simulink model "controller"  (Simulink 8.3)
settings: Solver=FixedStepDiscrete  StartTime=0.0  StopTime=inf  FixedStep=CONFIG.TS  RelTol=1e-3
InitFcn:
  | clc
  | cd(fileparts(which(bdroot)));
  | initTrqBalancingSeeSaw;
values from neighbouring files (symbols this model uses):
  LEFT_RIGHT_FOOT_IN_CONTACT = [1;1]    [initTrqBalancingSeeSaw.m]
undefined symbols (not defined in the file or in its folder): bVectorConstraints, CONFIG, ConstraintsMatrix, directionOfOscillation, DiscIntNeverNeededParam, gain, noOscillationTime, referenceParams, reg, ROBOT_DOF, sat, seesaw
undefined symbols (not defined in the file): FRAMES
libraries: WBToolboxLibrary x43
settings Model: Creator=makaveli  LastModifiedBy=gabri
settings DataIOCC: SignalLoggingSaveFormat=Dataset
settings DebuggingCC: UnderspecifiedInitializationDetection=Simplified  MergeDetectMultiDrivingBlocksExec=error  FrameProcessingCompatibilityMsg=error  StateNameClashWarn=none
settings GRTTargetCC: CombineOutputUpdateFcns=on  GRTInterface=off
settings ConfigComp: CovMetricSettings=dw  CovHtmlReporting=on  CovSaveCumulativeToWorkspaceVar=on  CovSaveSingleToWorkspaceVar=on  CovExternalEMLEnable=off  CovSFcnEnable=off

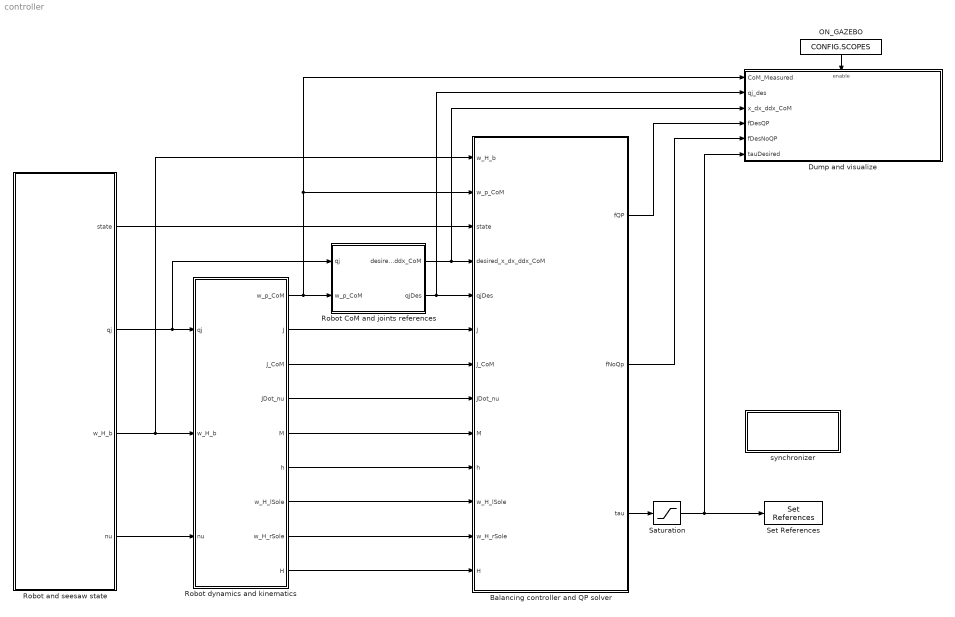
== system controller ==
  Balancing controller and QP solver : Subsystem
  Dump and visualize : Subsystem
  "ON_GAZEBO " : Constant  Value=CONFIG.SCOPES
  Robot CoM and joints references : Subsystem  Priority=2
  Robot and seesaw state : Subsystem
  Robot dynamics and kinematics : Subsystem  Priority=3
  Saturation : Saturate  UpperLimit=sat.torque  LowerLimit=-sat.torque
  Set References : WBToolboxLibrary/wholeBodyActuators/Set References  controlType=Torque  fullOrSubControl=Full  controlledJoints=''  robotName=WBT_robotName  localName=WBT_modelName  wbiFile=WBT_wbiFilename  wbiList=WBT_wbiList
  synchronizer : Subsystem
      mask Display: disp('SYNCHRONIZER')
  wires:
  Robot and seesaw state/1(state) -> Balancing controller and QP solver/3(state)
  Robot CoM and joints references/2(qjDes) -> Dump and visualize/2(qj_des), Balancing controller and QP solver/5(qjDes)
  Robot CoM and joints references/1(desired_x_dx_ddx_CoM) -> Dump and visualize/3(x_dx_ddx_CoM), Balancing controller and QP solver/4(desired_x_dx_ddx_CoM)
  Robot and seesaw state/4(nu) -> Robot dynamics and kinematics/3(nu)
  Robot and seesaw state/2(qj) -> Robot CoM and joints references/1(qj), Robot dynamics and kinematics/1(qj)
  Robot dynamics and kinematics/1(w_p_CoM) -> Balancing controller and QP solver/2(w_p_CoM), Dump and visualize/1(CoM_Measured), Robot CoM and joints references/2(w_p_CoM)
  Robot dynamics and kinematics/2("J ") -> Balancing controller and QP solver/6(J)
  Robot dynamics and kinematics/3(J_CoM) -> Balancing controller and QP solver/7(J_CoM)
  Robot dynamics and kinematics/4(JDot_nu) -> Balancing controller and QP solver/8(JDot_nu)
  Robot dynamics and kinematics/5(M) -> Balancing controller and QP solver/9(M)
  Robot dynamics and kinematics/6(h) -> Balancing controller and QP solver/10(h)
  Robot dynamics and kinematics/7(w_H_lSole) -> Balancing controller and QP solver/11(w_H_lSole)
  Robot dynamics and kinematics/8(w_H_rSole) -> Balancing controller and QP solver/12(w_H_rSole)
  Robot dynamics and kinematics/9(H) -> Balancing controller and QP solver/13(H)
  Balancing controller and QP solver/1(fQP) -> Dump and visualize/4(fDesQP)
  Balancing controller and QP solver/2(fNoQp) -> Dump and visualize/5(fDesNoQP)
  "ON_GAZEBO "/1 -> Dump and visualize/Enable
  Balancing controller and QP solver/3(tau) -> Saturation/1
  Saturation/1 -> Dump and visualize/6(tauDesired), Set References/1
  Robot and seesaw state/3(w_H_b) -> Balancing controller and QP solver/1(w_H_b), Robot dynamics and kinematics/2(w_H_b)

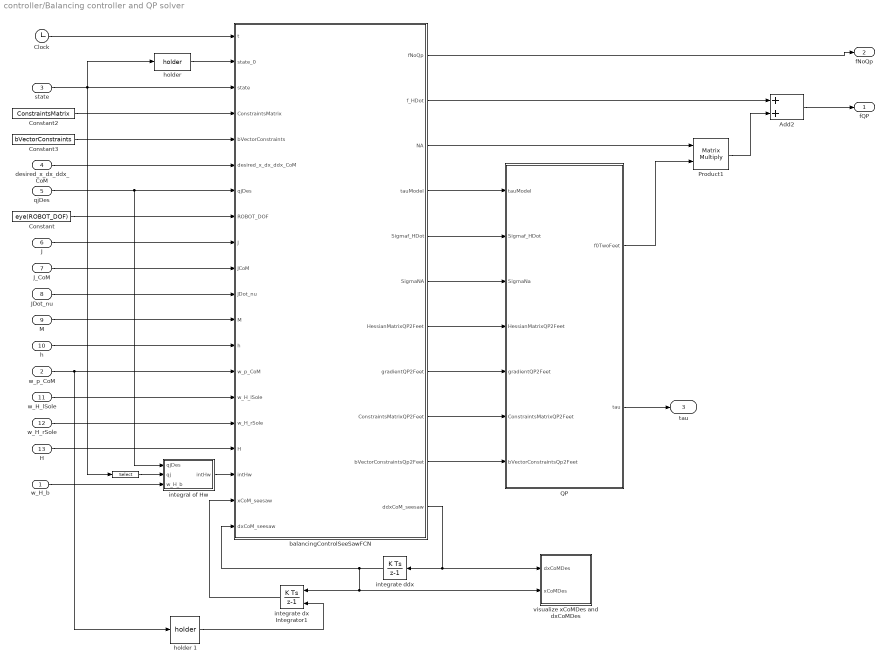
== system controller/Balancing controller and QP solver ==
  w_H_b : Inport
  w_p_CoM : Inport  Port=2
  state : Inport  Port=3
  desired_x_dx_ddx_CoM : Inport  Port=4
  qjDes : Inport  Port=5
  J : Inport  Port=6
  J_CoM : Inport  Port=7
  JDot_nu : Inport  Port=8
  M : Inport  Port=9
  h : Inport  Port=10
  w_H_lSole : Inport  Port=11
  w_H_rSole : Inport  Port=12
  H : Inport  Port=13
  " " : Selector  InputPortWidth=20+2*ROBOT_DOF  Indices=[12:11+ROBOT_DOF]
  Add2 : Sum
  Clock : Clock
  Constant : Constant  Value=eye(ROBOT_DOF)
  Constant2 : Constant  Value=ConstraintsMatrix
  Constant3 : Constant  Value=bVectorConstraints
  Product1 : Product  Multiplication=Matrix(*)
  QP : Subsystem
  balancingControlSeeSawFCN : MATLAB Function  TreatAsAtomicUnit=on
  "holder " : WBToolboxLibrary/Utilities/holder 
  holder 1 : WBToolboxLibrary/Utilities/holder 
  "integral of Hw " : Subsystem
  integrate ddx : DiscreteIntegrator  InitialCondition=zeros(3,1)  SampleTime=CONFIG.TS  ICPrevOutput=DiscIntNeverNeededParam  ICPrevScaledInput=DiscIntNeverNeededParam
  integrate dx Integrator1 : DiscreteIntegrator  InitialConditionSource=external  InitialCondition=zeros(3,1)  SampleTime=CONFIG.TS  ICPrevOutput=DiscIntNeverNeededParam  ICPrevScaledInput=DiscIntNeverNeededParam
  visualize xCoMDes and dxCoMDes : Subsystem
  fQP : Outport
  fNoQp : Outport  Port=2
  tau : Outport  Port=3
  wires:
  Clock/1 -> balancingControlSeeSawFCN/1(t)
  Constant/1 -> balancingControlSeeSawFCN/8(ROBOT_DOF)
  Constant2/1 -> balancingControlSeeSawFCN/4(ConstraintsMatrix)
  Constant3/1 -> balancingControlSeeSawFCN/5(bVectorConstraints)
  QP/1(f0TwoFeet) -> Product1/2
  balancingControlSeeSawFCN/9(ConstraintsMatrixQP2Feet) -> QP/6(ConstraintsMatrixQP2Feet)
  QP/2(tau) -> tau/1
  balancingControlSeeSawFCN/1(fNoQp) -> fNoQp/1
  Product1/1 -> Add2/2
  balancingControlSeeSawFCN/3(NA) -> Product1/1
  balancingControlSeeSawFCN/2(f_HDot) -> Add2/1
  Add2/1 -> fQP/1
  "integral of Hw "/1(intHw) -> balancingControlSeeSawFCN/18(intHw)
  balancingControlSeeSawFCN/4(tauModel) -> QP/1(tauModel)
  balancingControlSeeSawFCN/5(Sigmaf_HDot) -> QP/2(Sigmaf_HDot)
  balancingControlSeeSawFCN/6(SigmaNA) -> QP/3(SigmaNa)
  balancingControlSeeSawFCN/7(HessianMatrixQP2Feet) -> QP/4(HessianMatrixQP2Feet)
  balancingControlSeeSawFCN/8(gradientQP2Feet) -> QP/5(gradientQP2Feet)
  balancingControlSeeSawFCN/10(bVectorConstraintsQp2Feet) -> QP/7(bVectorConstraintsQp2Feet)
  state/1 -> " "/1, balancingControlSeeSawFCN/3(state), "holder "/1
  desired_x_dx_ddx_CoM/1 -> balancingControlSeeSawFCN/6(desired_x_dx_ddx_CoM)
  qjDes/1 -> "integral of Hw "/1(qjDes), balancingControlSeeSawFCN/7(qjDes)
  J/1 -> balancingControlSeeSawFCN/9(J)
  J_CoM/1 -> balancingControlSeeSawFCN/10(JCoM)
  JDot_nu/1 -> balancingControlSeeSawFCN/11(JDot_nu)
  M/1 -> balancingControlSeeSawFCN/12(M)
  h/1 -> balancingControlSeeSawFCN/13(h)
  w_H_lSole/1 -> balancingControlSeeSawFCN/15(w_H_lSole)
  w_H_rSole/1 -> balancingControlSeeSawFCN/16(w_H_rSole)
  H/1 -> balancingControlSeeSawFCN/17(H)
  w_p_CoM/1 -> balancingControlSeeSawFCN/14(w_p_CoM), holder 1/1
  "holder "/1 -> balancingControlSeeSawFCN/2(state_0)
  w_H_b/1 -> "integral of Hw "/3(w_H_b)
  " "/1 -> "integral of Hw "/2(qj)
  balancingControlSeeSawFCN/11(ddxCoM_seesaw) -> integrate ddx/1, visualize xCoMDes and dxCoMDes/1(dxCoMDes)
  integrate dx Integrator1/1 -> balancingControlSeeSawFCN/19(xCoM_seesaw)
  integrate ddx/1 -> integrate dx Integrator1/1, visualize xCoMDes and dxCoMDes/2(xCoMDes), balancingControlSeeSawFCN/20(dxCoM_seesaw)
  holder 1/1 -> integrate dx Integrator1/2

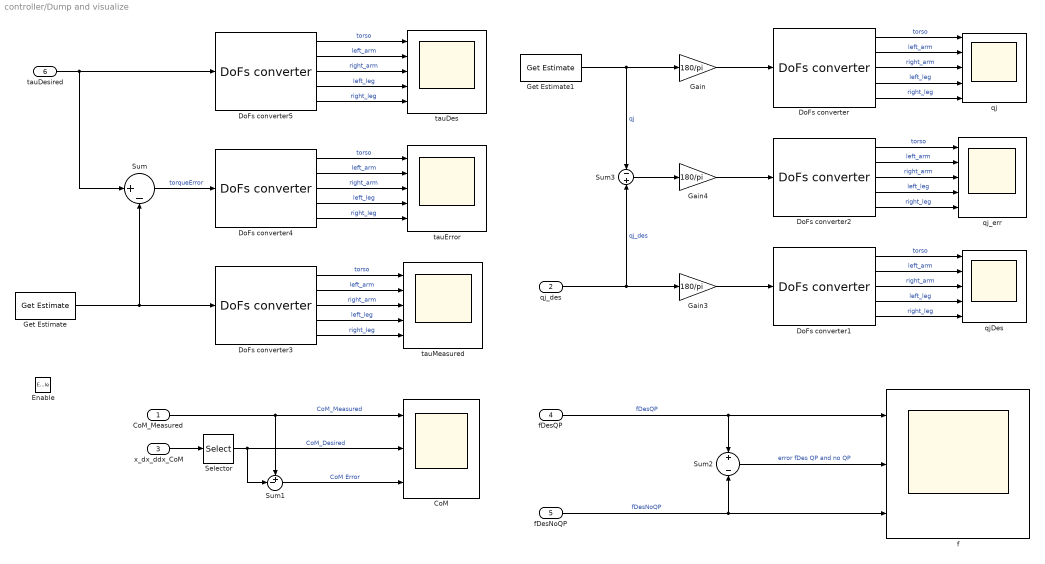
== system controller/Dump and visualize ==
  CoM_Measured : Inport
  qj_des : Inport  Port=2
  x_dx_ddx_CoM : Inport  Port=3
  fDesQP : Inport  Port=4
  fDesNoQP : Inport  Port=5
  tauDesired : Inport  Port=6
  Enable : EnablePort
  CoM : Scope  NumInputPorts=3
      settings: YMin=-5~-5~-5  YMax=5~5~5
  DoFs converter{,1..5} (6 alike) : WBToolboxLibrary/Utilities/DoFs converter  yarp2WBIOption=From WBI to YARP  robotName=WBT_robotName  localName=WBT_modelName  wbiFile=WBT_wbiFilename  wbiList=WBT_wbiList
  Gain : Gain  Gain=180/pi
  Gain3 : Gain  Gain=180/pi
  Gain4 : Gain  Gain=180/pi
  Get Estimate : WBToolboxLibrary/wholeBodyStates/Get Estimate  estimateType=Joints Torque  robotName=WBT_robotName  localName=WBT_modelName  wbiFile=WBT_wbiFilename  wbiList=WBT_wbiList
  Get Estimate1 : WBToolboxLibrary/wholeBodyStates/Get Estimate  estimateType=Joints Position  robotName=WBT_robotName  localName=WBT_modelName  wbiFile=WBT_wbiFilename  wbiList=WBT_wbiList
  Selector : Selector  NumberOfDimensions=2  IndexOptions=Index vector (dialog),Index vector (dialog)  Indices=[1:3],1  OutputSizes=1,1
  Sum : Sum  Inputs=|+-
  Sum1 : Sum  Inputs=+-|
  Sum2 : Sum  Inputs=+|-
  Sum3 : Sum  Inputs=-|+
  f : Scope  NumInputPorts=3
      settings: YMin=-5~-5~-5  YMax=5~5~5
  qj : Scope  NumInputPorts=5
      settings: YMin=-5~-5~-5~-5~-5  YMax=5~5~5~5~5
  qjDes : Scope  NumInputPorts=5
      settings: YMin=-5~-5~-5~-5~-5  YMax=5~5~5~5~5
  qj_err : Scope  NumInputPorts=5
      settings: YMin=-5~-5~-5~-5~-5  YMax=5~5~5~5~5
  tauDes : Scope  NumInputPorts=5
      settings: YMin=-5~-5~-5~-5~-5  YMax=5~5~5~5~5
  tauError : Scope  NumInputPorts=5
      settings: YMin=-5~-5~-5~-5~-5  YMax=5~5~5~5~5
  tauMeasured : Scope  NumInputPorts=5
      settings: YMin=-5~-5~-5~-5~-5  YMax=5~5~5~5~5
  wires:
  x_dx_ddx_CoM/1 -> Selector/1
  CoM_Measured/1 -> Sum1/1, CoM/1  "CoM_Measured"
  Get Estimate1/1 -> Sum3/1, Gain/1  "qj"
  Gain/1 -> DoFs converter/1
  DoFs converter/5 -> qj/5  "right_leg"
  DoFs converter/1 -> qj/1  "torso"
  DoFs converter/2 -> qj/2  "left_arm"
  DoFs converter/4 -> qj/4  "left_leg"
  DoFs converter/3 -> qj/3  "right_arm"
  fDesQP/1 -> Sum2/1, f/1  "fDesQP"
  Sum2/1 -> f/2  "error fDes QP and no QP"
  fDesNoQP/1 -> Sum2/2, f/3  "fDesNoQP"
  tauDesired/1 -> DoFs converter5/1, Sum/1
  Get Estimate/1 -> Sum/2, DoFs converter3/1
  DoFs converter5/5 -> tauDes/5  "right_leg"
  DoFs converter5/1 -> tauDes/1  "torso"
  DoFs converter5/2 -> tauDes/2  "left_arm"
  DoFs converter5/4 -> tauDes/4  "left_leg"
  DoFs converter5/3 -> tauDes/3  "right_arm"
  DoFs converter4/5 -> tauError/5  "right_leg"
  DoFs converter4/1 -> tauError/1  "torso"
  DoFs converter4/2 -> tauError/2  "left_arm"
  DoFs converter4/4 -> tauError/4  "left_leg"
  DoFs converter4/3 -> tauError/3  "right_arm"
  Sum/1 -> DoFs converter4/1  "torqueError"
  DoFs converter3/5 -> tauMeasured/5  "right_leg"
  DoFs converter3/1 -> tauMeasured/1  "torso"
  DoFs converter3/2 -> tauMeasured/2  "left_arm"
  DoFs converter3/4 -> tauMeasured/4  "left_leg"
  DoFs converter3/3 -> tauMeasured/3  "right_arm"
  qj_des/1 -> Sum3/2, Gain3/1  "qj_des"
  Gain3/1 -> DoFs converter1/1
  DoFs converter1/5 -> qjDes/5  "right_leg"
  DoFs converter1/1 -> qjDes/1  "torso"
  DoFs converter1/2 -> qjDes/2  "left_arm"
  DoFs converter1/4 -> qjDes/4  "left_leg"
  DoFs converter1/3 -> qjDes/3  "right_arm"
  Gain4/1 -> DoFs converter2/1
  DoFs converter2/5 -> qj_err/5  "right_leg"
  DoFs converter2/1 -> qj_err/1  "torso"
  DoFs converter2/2 -> qj_err/2  "left_arm"
  DoFs converter2/4 -> qj_err/4  "left_leg"
  DoFs converter2/3 -> qj_err/3  "right_arm"
  Sum3/1 -> Gain4/1
  Selector/1 -> Sum1/2, CoM/2  "CoM_Desired"
  Sum1/1 -> CoM/3  "CoM Error"

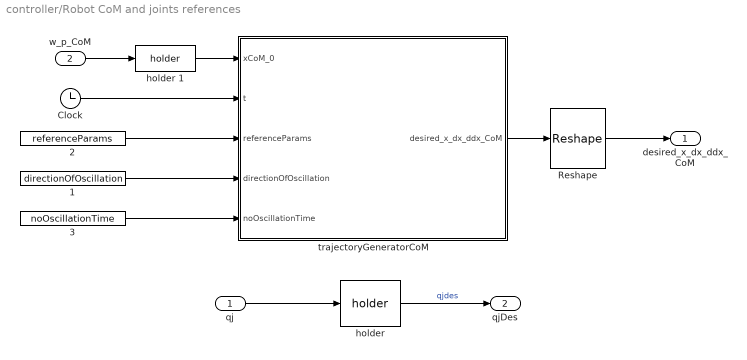
== system controller/Robot CoM and joints references ==
  qj : Inport
  w_p_CoM : Inport  Port=2
  "    1" : Constant  Value=directionOfOscillation
  "    2" : Constant  Value=referenceParams
  "    3" : Constant  Value=noOscillationTime
  Clock : Clock
  Reshape : Reshape  OutputDimensionality=Customize  OutputDimensions=[3,3]
  "holder " : WBToolboxLibrary/Utilities/holder 
  holder 1 : WBToolboxLibrary/Utilities/holder 
  trajectoryGeneratorCoM : MATLAB Function  TreatAsAtomicUnit=on
  desired_x_dx_ddx_CoM : Outport
  qjDes : Outport  Port=2
  wires:
  qj/1 -> "holder "/1
  "holder "/1 -> qjDes/1  "qjdes"
  holder 1/1 -> trajectoryGeneratorCoM/1(xCoM_0)
  "    2"/1 -> trajectoryGeneratorCoM/3(referenceParams)
  Clock/1 -> trajectoryGeneratorCoM/2(t)
  "    1"/1 -> trajectoryGeneratorCoM/4(directionOfOscillation)
  "    3"/1 -> trajectoryGeneratorCoM/5(noOscillationTime)
  trajectoryGeneratorCoM/1(desired_x_dx_ddx_CoM) -> Reshape/1
  Reshape/1 -> desired_x_dx_ddx_CoM/1
  w_p_CoM/1 -> holder 1/1

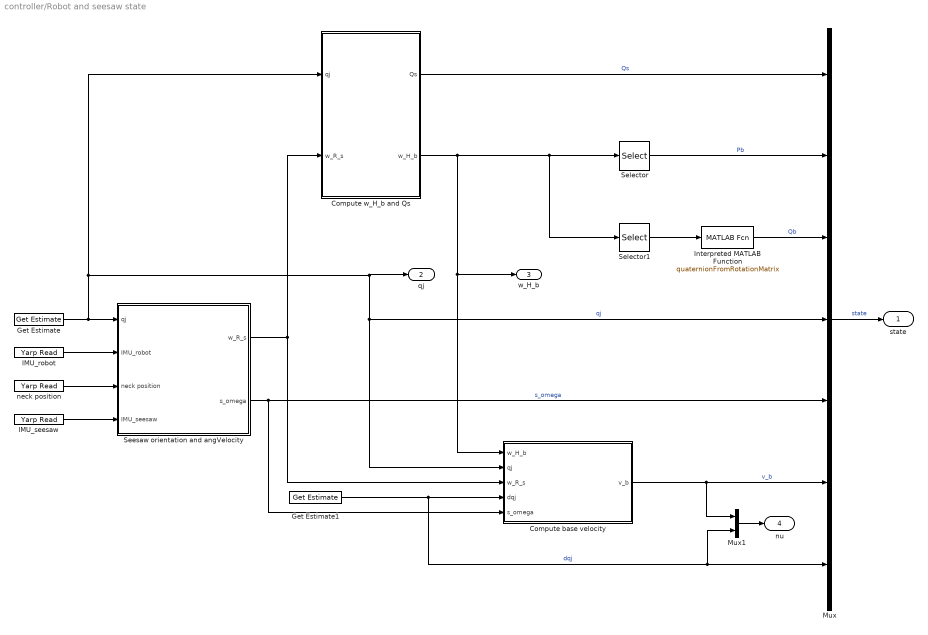
== system controller/Robot and seesaw state ==
  Compute base velocity : Subsystem
  "Compute w_H_b and Qs " : Subsystem
  Get Estimate : WBToolboxLibrary/wholeBodyStates/Get Estimate  estimateType=Joints Position  robotName=WBT_robotName  localName=WBT_modelName  wbiFile=WBT_wbiFilename  wbiList=WBT_wbiList
  Get Estimate1 : WBToolboxLibrary/wholeBodyStates/Get Estimate  estimateType=Joints Velocity  robotName=WBT_robotName  localName=WBT_modelName  wbiFile=WBT_wbiFilename  wbiList=WBT_wbiList
  IMU_robot : WBToolboxLibrary/Utilities/Yarp Read  portName=PORTS.IMU  signalSize=12  blocking=off  timestamp=off  autoconnect=on  errorOnConnection=on
  IMU_seesaw : WBToolboxLibrary/Utilities/Yarp Read  portName=PORTS.IMU_SEESAW  signalSize=12  blocking=off  timestamp=off  autoconnect=on  errorOnConnection=off
  Interpreted MATLAB Function : MATLABFcn  MATLABFcn=quaternionFromRotationMatrix  OutputDimensions=4
  Mux : Mux  Inputs=7
  Mux1 : Mux  Inputs=2
  Seesaw orientation and angVelocity : Subsystem
  Selector : Selector  NumberOfDimensions=2  InputPortWidth=3  IndexOptions=Index vector (dialog),Index vector (dialog)  Indices=[1:3],4  OutputSizes=1,1
  Selector1 : Selector  NumberOfDimensions=2  InputPortWidth=3  IndexOptions=Index vector (dialog),Index vector (dialog)  Indices=[1:3],[1:3]  OutputSizes=1,1
  neck position : WBToolboxLibrary/Utilities/Yarp Read  portName=PORTS.NECK  signalSize=6  blocking=off  timestamp=off  autoconnect=on  errorOnConnection=on
  state : Outport
  qj : Outport  Port=2
  w_H_b : Outport  Port=3
  nu : Outport  Port=4
  wires:
  IMU_robot/1 -> Seesaw orientation and angVelocity/2(IMU_robot)
  IMU_seesaw/1 -> Seesaw orientation and angVelocity/4(IMU_seesaw)
  neck position/1 -> Seesaw orientation and angVelocity/3(neck position)
  Mux/1 -> state/1  "state"
  Selector/1 -> Mux/2  "Pb"
  Selector1/1 -> Interpreted MATLAB Function/1
  Interpreted MATLAB Function/1 -> Mux/3  "Qb"
  Get Estimate/1 -> "Compute w_H_b and Qs "/1(qj), qj/1, Compute base velocity/2(qj), Mux/4, Seesaw orientation and angVelocity/1(qj)  "qj"
  Mux1/1 -> nu/1
  Compute base velocity/1(v_b) -> Mux1/1, Mux/6  "v_b"
  Seesaw orientation and angVelocity/1(w_R_s) -> "Compute w_H_b and Qs "/2(w_R_s), Compute base velocity/3(w_R_s)
  Seesaw orientation and angVelocity/2(s_omega) -> Mux/5, Compute base velocity/5(s_omega)  "s_omega"
  Get Estimate1/1 -> Mux1/2, Mux/7, Compute base velocity/4(dqj)  "dqj"
  "Compute w_H_b and Qs "/2(w_H_b) -> w_H_b/1, Compute base velocity/1(w_H_b), Selector1/1, Selector/1
  "Compute w_H_b and Qs "/1(Qs) -> Mux/1  "Qs"

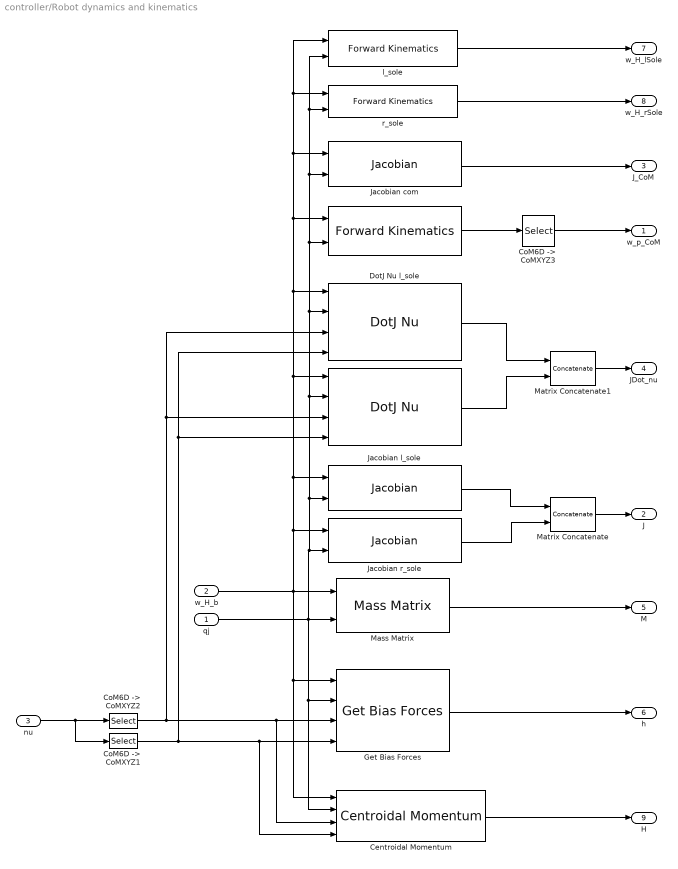
== system controller/Robot dynamics and kinematics ==
  qj : Inport
  w_H_b : Inport  Port=2
  nu : Inport  Port=3
  " " : WBToolboxLibrary/wholeBodyModel/Kinematics/Forward Kinematics  frameName='com'  robotName=WBT_robotName  localName=WBT_modelName  wbiFile=WBT_wbiFilename  wbiList=WBT_wbiList
  "  " : WBToolboxLibrary/wholeBodyModel/Jacobians/DotJ Nu  frameName='r_sole'  robotName=WBT_robotName  localName=WBT_modelName  wbiFile=WBT_wbiFilename  wbiList=WBT_wbiList
  Centroidal Momentum : WBToolboxLibrary/wholeBodyModel/Dynamics/Centroidal Momentum  robotName=WBT_robotName  localName=WBT_modelName  wbiFile=WBT_wbiFilename  wbiList=WBT_wbiList
  "CoM6D ->  CoMXYZ1" : Selector  InputPortWidth=6+ROBOT_DOF  Indices=[7:6+ROBOT_DOF]
  "CoM6D ->  CoMXYZ2" : Selector  InputPortWidth=6+ROBOT_DOF  Indices=[1 2 3 4 5 6]
  "CoM6D ->  CoMXYZ3" : Selector  NumberOfDimensions=2  InputPortWidth=7  IndexOptions=Index vector (dialog),Index vector (dialog)  Indices=[1 2 3],[4]  OutputSizes=1,1
  "DotJ Nu l_sole " : WBToolboxLibrary/wholeBodyModel/Jacobians/DotJ Nu  frameName='l_sole'  robotName=WBT_robotName  localName=WBT_modelName  wbiFile=WBT_wbiFilename  wbiList=WBT_wbiList
  Get Bias Forces : WBToolboxLibrary/wholeBodyModel/Dynamics/Get Bias Forces  robotName=WBT_robotName  localName=WBT_modelName  wbiFile=WBT_wbiFilename  wbiList=WBT_wbiList  explicitGravity=off
  Jacobian com : WBToolboxLibrary/wholeBodyModel/Jacobians/Jacobian  frameName='com'  robotName=WBT_robotName  localName=WBT_modelName  wbiFile=WBT_wbiFilename  wbiList=WBT_wbiList
  Jacobian l_sole : WBToolboxLibrary/wholeBodyModel/Jacobians/Jacobian  frameName='l_sole'  robotName=WBT_robotName  localName=WBT_modelName  wbiFile=WBT_wbiFilename  wbiList=WBT_wbiList
  Jacobian r_sole : WBToolboxLibrary/wholeBodyModel/Jacobians/Jacobian  frameName='r_sole'  robotName=WBT_robotName  localName=WBT_modelName  wbiFile=WBT_wbiFilename  wbiList=WBT_wbiList
  Mass Matrix : WBToolboxLibrary/wholeBodyModel/Dynamics/Mass Matrix  robotName=WBT_robotName  localName=WBT_modelName  wbiFile=WBT_wbiFilename  wbiList=WBT_wbiList
  Matrix Concatenate : Concatenate  Mode=Multidimensional array
  Matrix Concatenate1 : Concatenate  Mode=Multidimensional array
  l_sole : WBToolboxLibrary/wholeBodyModel/Kinematics/Forward Kinematics  frameName='l_sole'  robotName=WBT_robotName  localName=WBT_modelName  wbiFile=WBT_wbiFilename  wbiList=WBT_wbiList
  r_sole : WBToolboxLibrary/wholeBodyModel/Kinematics/Forward Kinematics  frameName='r_sole'  robotName=WBT_robotName  localName=WBT_modelName  wbiFile=WBT_wbiFilename  wbiList=WBT_wbiList
  w_p_CoM : Outport
  "J " : Outport  Port=2
  J_CoM : Outport  Port=3
  JDot_nu : Outport  Port=4
  M : Outport  Port=5
  h : Outport  Port=6
  w_H_lSole : Outport  Port=7
  w_H_rSole : Outport  Port=8
  H : Outport  Port=9
  wires:
  Get Bias Forces/1 -> h/1
  Matrix Concatenate1/1 -> JDot_nu/1
  Jacobian r_sole/1 -> Matrix Concatenate/2
  l_sole/1 -> w_H_lSole/1
  r_sole/1 -> w_H_rSole/1
  Matrix Concatenate/1 -> "J "/1
  Jacobian l_sole/1 -> Matrix Concatenate/1
  Jacobian com/1 -> J_CoM/1
  w_H_b/1 -> Jacobian r_sole/1, "  "/1, " "/1, r_sole/1, l_sole/1, Jacobian com/1, "DotJ Nu l_sole "/1, Jacobian l_sole/1, Mass Matrix/1, Centroidal Momentum/1, Get Bias Forces/1
  qj/1 -> Centroidal Momentum/2, Get Bias Forces/2, r_sole/2, l_sole/2, Jacobian com/2, " "/2, "DotJ Nu l_sole "/2, "  "/2, Jacobian l_sole/2, Jacobian r_sole/2, Mass Matrix/2
  "CoM6D ->  CoMXYZ2"/1 -> "  "/3, "DotJ Nu l_sole "/3, Centroidal Momentum/3, Get Bias Forces/3
  "CoM6D ->  CoMXYZ1"/1 -> Centroidal Momentum/4, Get Bias Forces/4, "  "/4, "DotJ Nu l_sole "/4
  nu/1 -> "CoM6D ->  CoMXYZ1"/1, "CoM6D ->  CoMXYZ2"/1
  Centroidal Momentum/1 -> H/1
  Mass Matrix/1 -> M/1
  "DotJ Nu l_sole "/1 -> Matrix Concatenate1/1
  "  "/1 -> Matrix Concatenate1/2
  "CoM6D ->  CoMXYZ3"/1 -> w_p_CoM/1
  " "/1 -> "CoM6D ->  CoMXYZ3"/1

== system controller/synchronizer ==
  GAZEBO_SYNCHRONIZER : Subsystem
  Logical Operator : Logic  Operator=NOT  AllPortsSameDT=off  OutDataTypeStr=boolean
  "ON_GAZEBO " : Constant  Value=CONFIG.ON_GAZEBO
  REAL_TIME_SYNC : Subsystem
  wires:
  Logical Operator/1 -> REAL_TIME_SYNC/Enable
  "ON_GAZEBO "/1 -> Logical Operator/1, GAZEBO_SYNCHRONIZER/Enable

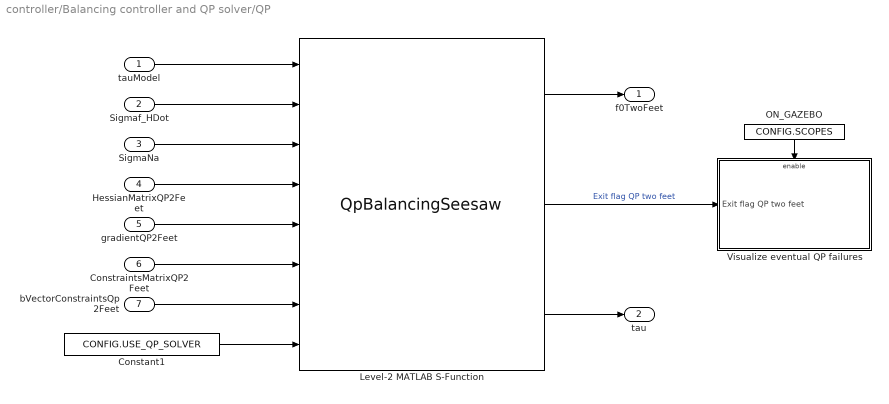
== system controller/Balancing controller and QP solver/QP ==
  tauModel : Inport
  Sigmaf_HDot : Inport  Port=2
  SigmaNa : Inport  Port=3
  HessianMatrixQP2Feet : Inport  Port=4
  gradientQP2Feet : Inport  Port=5
  ConstraintsMatrixQP2Feet : Inport  Port=6
  bVectorConstraintsQp2Feet : Inport  Port=7
  Constant1 : Constant  Value=CONFIG.USE_QP_SOLVER
  Level-2 MATLAB S-Function : M-S-Function  FunctionName=QpBalancingSeesaw
  "ON_GAZEBO " : Constant  Value=CONFIG.SCOPES
  Visualize eventual QP failures : Subsystem
  f0TwoFeet : Outport
  tau : Outport  Port=2
  wires:
  Level-2 MATLAB S-Function/1 -> f0TwoFeet/1
  Level-2 MATLAB S-Function/2 -> Visualize eventual QP failures/1(Exit flag QP two feet)  "Exit flag QP two feet"
  "ON_GAZEBO "/1 -> Visualize eventual QP failures/Enable
  Constant1/1 -> Level-2 MATLAB S-Function/8
  HessianMatrixQP2Feet/1 -> Level-2 MATLAB S-Function/4
  gradientQP2Feet/1 -> Level-2 MATLAB S-Function/5
  ConstraintsMatrixQP2Feet/1 -> Level-2 MATLAB S-Function/6
  bVectorConstraintsQp2Feet/1 -> Level-2 MATLAB S-Function/7
  tauModel/1 -> Level-2 MATLAB S-Function/1
  Sigmaf_HDot/1 -> Level-2 MATLAB S-Function/2
  SigmaNa/1 -> Level-2 MATLAB S-Function/3
  Level-2 MATLAB S-Function/3 -> tau/1

== system controller/Balancing controller and QP solver/integral of Hw  ==
  qjDes : Inport
  qj : Inport  Port=2
  w_H_b : Inport  Port=3
  "  " : WBToolboxLibrary/wholeBodyModel/Jacobians/Jacobian  frameName='r_sole'  robotName=WBT_robotName  localName=WBT_modelName  wbiFile=WBT_wbiFilename  wbiList=WBT_wbiList
  Centroidal Momentum : WBToolboxLibrary/wholeBodyModel/Dynamics/Centroidal Momentum  robotName=WBT_robotName  localName=WBT_modelName  wbiFile=WBT_wbiFilename  wbiList=WBT_wbiList
  Constant4 : Constant  Value=LEFT_RIGHT_FOOT_IN_CONTACT
  Jacobian : WBToolboxLibrary/wholeBodyModel/Jacobians/Jacobian  frameName='l_sole'  robotName=WBT_robotName  localName=WBT_modelName  wbiFile=WBT_wbiFilename  wbiList=WBT_wbiList
  MATLAB Function : MATLAB Function  TreatAsAtomicUnit=on
  Selector : Selector  InputPortWidth=6  Indices=[4 5 6]
  Sum : Sum  Inputs=|-+
  "holder " : WBToolboxLibrary/Utilities/holder 
  intHw : Outport
  wires:
  qjDes/1 -> Sum/1, "  "/2, Jacobian/2, Centroidal Momentum/2
  qj/1 -> Sum/2
  Sum/1 -> MATLAB Function/1(qjErr), Centroidal Momentum/4
  MATLAB Function/1(vbEquivalent) -> Centroidal Momentum/3
  Jacobian/1 -> MATLAB Function/2(JL)
  Centroidal Momentum/1 -> Selector/1
  Selector/1 -> intHw/1
  "  "/1 -> MATLAB Function/3(JR)
  w_H_b/1 -> "holder "/1
  Constant4/1 -> MATLAB Function/4(activeFeetConstraints)
  "holder "/1 -> Centroidal Momentum/1, Jacobian/1, "  "/1

== system controller/Balancing controller and QP solver/visualize xCoMDes and dxCoMDes ==
  dxCoMDes : Inport
  xCoMDes : Inport  Port=2
  vis_dxCoMDes : Scope
      settings: SaveName=ScopeData12
  vis_xCoMDes : Scope
      settings: YMin=-0.011  YMax=0.007  SaveName=ScopeData11
  wires:
  dxCoMDes/1 -> vis_dxCoMDes/1
  xCoMDes/1 -> vis_xCoMDes/1

== system controller/Robot and seesaw state/Compute base velocity ==
  w_H_b : Inport
  qj : Inport  Port=2
  w_R_s : Inport  Port=3
  dqj : Inport  Port=4
  s_omega : Inport  Port=5
  Base and joints velocity : Subsystem
  Jacobian fixedLink : WBToolboxLibrary/wholeBodyModel/Jacobians/Jacobian  frameName=FRAMES.fixedLink  robotName=WBT_robotName  localName=WBT_modelName  wbiFile=WBT_wbiFilename  wbiList=WBT_wbiList
  "ON_GAZEBO " : Constant  Value=CONFIG.SCOPES
  evaluateBaseVelocity : MATLAB Function  Priority=10  TreatAsAtomicUnit=on
  v_b : Outport
  wires:
  w_R_s/1 -> evaluateBaseVelocity/2(w_R_s)
  w_H_b/1 -> Jacobian fixedLink/1
  evaluateBaseVelocity/1(v_base) -> Base and joints velocity/1(v_b), v_b/1
  s_omega/1 -> evaluateBaseVelocity/4(s_omega)
  qj/1 -> Jacobian fixedLink/2
  dqj/1 -> evaluateBaseVelocity/3(dqj), Base and joints velocity/2(dqj)
  Jacobian fixedLink/1 -> evaluateBaseVelocity/1(J_fixedLink)
  "ON_GAZEBO "/1 -> Base and joints velocity/Enable

== system controller/Robot and seesaw state/Compute w_H_b and Qs  ==
  qj : Inport
  w_R_s : Inport  Port=2
  Compute w_H_fixedLink : Subsystem
  MATLAB Function : MATLAB Function  Priority=10  TreatAsAtomicUnit=on
  Product1 : Product  Priority=19  Multiplication=Matrix(*)
  fixedLink_H_b : Subsystem  mask{link_name=FRAMES.fixedLink}
      mask prompts: link_name "link name"
      mask help:
      | This block evaluates the homogeneous transformation between the world and the root link, i.e. ^wH_b. It assumes that the link specified by the variable 'link_name' has a constant position
      | w.r.t. an inertial frame, but it can rotate arbitrarily. This rotation is retrived from the IMU sensor.
      mask Display:
      | str = strrep(link_name, '_','\_');
      | port_label('output',1,['{}^{',str '}H_{root}'],'texmode','on')
      | clear str;
      | 
      | port_label('input',1,'q_j','texmode','on')
  Qs : Outport
  w_H_b : Outport  Port=2
  wires:
  qj/1 -> fixedLink_H_b/1(qj)
  w_R_s/1 -> Compute w_H_fixedLink/1(w_R_s), MATLAB Function/1(w_R_s)
  fixedLink_H_b/1(link_H_root) -> Product1/2
  MATLAB Function/1(Qs) -> Qs/1  "Qs"
  Product1/1 -> w_H_b/1  "w_H_b"
  Compute w_H_fixedLink/1(w_H_fixedLink) -> Product1/1

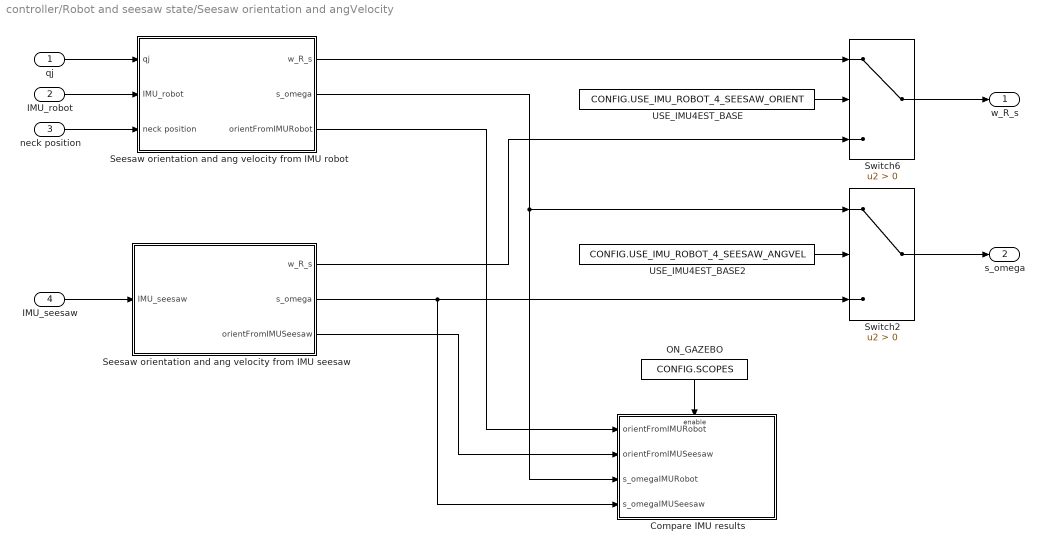
== system controller/Robot and seesaw state/Seesaw orientation and angVelocity ==
  qj : Inport
  IMU_robot : Inport  Port=2
  neck position : Inport  Port=3
  IMU_seesaw : Inport  Port=4
  Compare IMU results : Subsystem
  "ON_GAZEBO " : Constant  Value=CONFIG.SCOPES
  Seesaw orientation and ang velocity from IMU robot : Subsystem
  Seesaw orientation and ang velocity from IMU seesaw : Subsystem
  Switch2 : Switch  Criteria=u2 > Threshold
  Switch6 : Switch  Criteria=u2 > Threshold
  USE_IMU4EST_BASE : Constant  Value=CONFIG.USE_IMU_ROBOT_4_SEESAW_ORIENT
  USE_IMU4EST_BASE2 : Constant  Value=CONFIG.USE_IMU_ROBOT_4_SEESAW_ANGVEL
  w_R_s : Outport
  s_omega : Outport  Port=2
  wires:
  USE_IMU4EST_BASE/1 -> Switch6/2
  Switch6/1 -> w_R_s/1
  Seesaw orientation and ang velocity from IMU seesaw/1(w_R_s) -> Switch6/3
  IMU_seesaw/1 -> Seesaw orientation and ang velocity from IMU seesaw/1(IMU_seesaw)
  Seesaw orientation and ang velocity from IMU robot/1(w_R_s) -> Switch6/1
  neck position/1 -> Seesaw orientation and ang velocity from IMU robot/3(neck position)
  USE_IMU4EST_BASE2/1 -> Switch2/2
  IMU_robot/1 -> Seesaw orientation and ang velocity from IMU robot/2(IMU_robot)
  qj/1 -> Seesaw orientation and ang velocity from IMU robot/1(qj)
  Seesaw orientation and ang velocity from IMU robot/2(s_omega) -> Compare IMU results/3(s_omegaIMURobot), Switch2/1
  Seesaw orientation and ang velocity from IMU seesaw/2(s_omega) -> Compare IMU results/4(s_omegaIMUSeesaw), Switch2/3
  Switch2/1 -> s_omega/1
  Seesaw orientation and ang velocity from IMU robot/3(orientFromIMURobot) -> Compare IMU results/1(orientFromIMURobot)
  Seesaw orientation and ang velocity from IMU seesaw/3(orientFromIMUSeesaw) -> Compare IMU results/2(orientFromIMUSeesaw)
  "ON_GAZEBO "/1 -> Compare IMU results/Enable

== system controller/synchronizer/GAZEBO_SYNCHRONIZER ==
  Enable : EnablePort
  Simulator Synchronizer : WBToolboxLibrary/Utilities/Simulator Synchronizer  period=CONFIG.TS  serverPortName='/clock/rpc'  clientPortName='/WBT_synchronizer/rpc:o'

== system controller/synchronizer/REAL_TIME_SYNC ==
  Enable : EnablePort
  Real Time Synchronizer : WBToolboxLibrary/Utilities/Real Time Synchronizer  period=CONFIG.TS

== system controller/Balancing controller and QP solver/QP/Visualize eventual QP failures ==
  Exit flag QP two feet : Inport
  Enable : EnablePort
  "QP status (0: no failure, 1: not using)" : Scope
  wires:
  Exit flag QP two feet/1 -> "QP status (0: no failure, 1: not using)"/1

== system controller/Robot and seesaw state/Compute base velocity/Base and joints velocity ==
  v_b : Inport
  dqj : Inport  Port=2
  Enable : EnablePort
  DoFs converter : WBToolboxLibrary/Utilities/DoFs converter  yarp2WBIOption=From WBI to YARP  robotName=WBT_robotName  localName=WBT_modelName  wbiFile=WBT_wbiFilename  wbiList=WBT_wbiList
  dq_j : Scope  NumInputPorts=5
      settings: YMin=-5~-5~-5~-5~-5  YMax=5~5~5~5~5  SaveName=ScopeData2
  vb : Scope
      settings: SaveName=ScopeData10
  wires:
  DoFs converter/5 -> dq_j/5  "right_leg"
  DoFs converter/1 -> dq_j/1  "torso"
  DoFs converter/2 -> dq_j/2  "left_arm"
  DoFs converter/4 -> dq_j/4  "left_leg"
  DoFs converter/3 -> dq_j/3  "right_arm"
  dqj/1 -> DoFs converter/1
  v_b/1 -> vb/1

== system controller/Robot and seesaw state/Compute w_H_b and Qs /Compute w_H_fixedLink ==
  w_R_s : Inport
  fixedLink w.r.t the world frame : MATLAB Function  TreatAsAtomicUnit=on
  w_H_fixedLink : Outport
  wires:
  w_R_s/1 -> fixedLink w.r.t the world frame/1(w_R_s)
  fixedLink w.r.t the world frame/1(w_H_fixedLink) -> w_H_fixedLink/1

== system controller/Robot and seesaw state/Compute w_H_b and Qs /fixedLink_H_b ==
  qj : Inport
  Constant2 : Constant  Value=eye(4)
  Constant6 : Constant  Value=eye(4)
  Inv\*1 : Product  Inputs=/*  Multiplication=Matrix(*)
  link : WBToolboxLibrary/wholeBodyModel/Kinematics/Forward Kinematics  frameName=link_name  robotName=WBT_robotName  localName=WBT_modelName  wbiFile=WBT_wbiFilename  wbiList=WBT_wbiList
  root_link : WBToolboxLibrary/wholeBodyModel/Kinematics/Forward Kinematics  frameName='root_link'  robotName=WBT_robotName  localName=WBT_modelName  wbiFile=WBT_wbiFilename  wbiList=WBT_wbiList
  link_H_root : Outport
  wires:
  Constant6/1 -> link/1
  Inv\*1/1 -> link_H_root/1
  link/1 -> Inv\*1/1
  Constant2/1 -> root_link/1
  qj/1 -> root_link/2, link/2
  root_link/1 -> Inv\*1/2

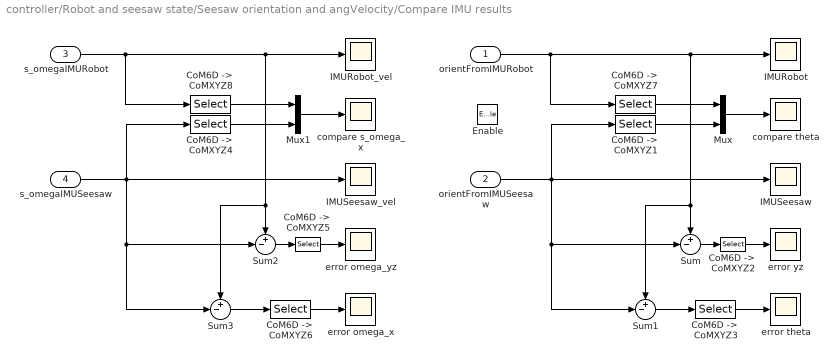
== system controller/Robot and seesaw state/Seesaw orientation and angVelocity/Compare IMU results ==
  orientFromIMURobot : Inport
  orientFromIMUSeesaw : Inport  Port=2
  s_omegaIMURobot : Inport  Port=3
  s_omegaIMUSeesaw : Inport  Port=4
  Enable : EnablePort
  CoM6D ->  CoMXYZ{1,3..4,6..8} (6 alike) : Selector  InputPortWidth=3  Indices=[1]
  "CoM6D ->  CoMXYZ2" : Selector  InputPortWidth=3  Indices=[2 3]
  "CoM6D ->  CoMXYZ5" : Selector  InputPortWidth=3  Indices=[2 3]
  IMURobot : Scope
  IMURobot_vel : Scope
      settings: SaveName=ScopeData5
  IMUSeesaw : Scope
  IMUSeesaw_vel : Scope
      settings: SaveName=ScopeData6
  Mux : Mux  Inputs=2
  Mux1 : Mux  Inputs=2
  Sum{,1..3} (4 alike) : Sum  Inputs=+-|
  compare s_omega_x : Scope
      settings: SaveName=ScopeData7
  compare theta : Scope
  error omega_x : Scope
      settings: SaveName=ScopeData8
  error omega_yz : Scope
      settings: SaveName=ScopeData9
  error theta : Scope
      settings: SaveName=ScopeData4
  error yz : Scope
      settings: SaveName=ScopeData3
  wires:
  orientFromIMURobot/1 -> "CoM6D ->  CoMXYZ7"/1, Sum1/1, Sum/1, IMURobot/1
  orientFromIMUSeesaw/1 -> Sum/2, Sum1/2, "CoM6D ->  CoMXYZ1"/1, IMUSeesaw/1
  Mux/1 -> compare theta/1
  "CoM6D ->  CoMXYZ1"/1 -> Mux/2
  "CoM6D ->  CoMXYZ7"/1 -> Mux/1
  Sum1/1 -> "CoM6D ->  CoMXYZ3"/1
  Sum/1 -> "CoM6D ->  CoMXYZ2"/1
  "CoM6D ->  CoMXYZ2"/1 -> error yz/1
  "CoM6D ->  CoMXYZ3"/1 -> error theta/1
  s_omegaIMURobot/1 -> "CoM6D ->  CoMXYZ8"/1, Sum3/1, Sum2/1, IMURobot_vel/1
  s_omegaIMUSeesaw/1 -> Sum2/2, Sum3/2, "CoM6D ->  CoMXYZ4"/1, IMUSeesaw_vel/1
  Mux1/1 -> compare s_omega_x/1
  "CoM6D ->  CoMXYZ4"/1 -> Mux1/2
  "CoM6D ->  CoMXYZ8"/1 -> Mux1/1
  Sum3/1 -> "CoM6D ->  CoMXYZ6"/1
  Sum2/1 -> "CoM6D ->  CoMXYZ5"/1
  "CoM6D ->  CoMXYZ5"/1 -> error omega_yz/1
  "CoM6D ->  CoMXYZ6"/1 -> error omega_x/1

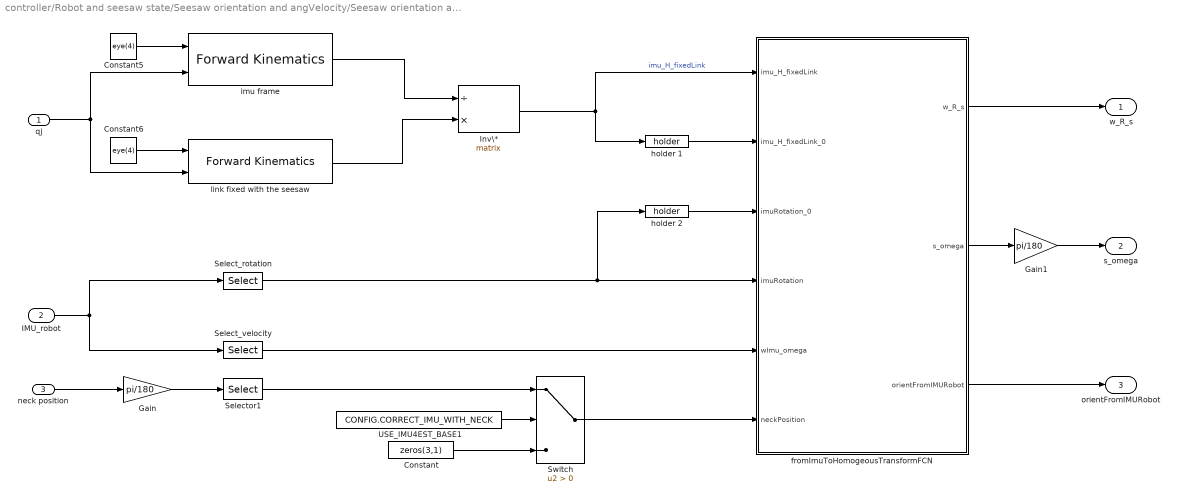
== system controller/Robot and seesaw state/Seesaw orientation and angVelocity/Seesaw orientation and ang velocity from IMU robot ==
  qj : Inport
  IMU_robot : Inport  Port=2
  neck position : Inport  Port=3
  Constant : Constant  Value=zeros(3,1)
  Constant5 : Constant  Value=eye(4)
  Constant6 : Constant  Value=eye(4)
  Gain : Gain  Gain=pi/180
  Gain1 : Gain  Gain=pi/180
  Inv\* : Product  Inputs=/*  Multiplication=Matrix(*)
  Select_rotation : Selector  InputPortWidth=12  Indices=[1 2 3]
  Select_velocity : Selector  InputPortWidth=12  Indices=[7 8 9]
  Selector1 : Selector  InputPortWidth=6  Indices=[1:3]
  Switch : Switch  Criteria=u2 > Threshold
  USE_IMU4EST_BASE1 : Constant  Value=CONFIG.CORRECT_IMU_WITH_NECK
  fromImuToHomogeousTransformFCN : MATLAB Function  TreatAsAtomicUnit=on
  holder 1 : WBToolboxLibrary/Utilities/holder 
  holder 2 : WBToolboxLibrary/Utilities/holder 
  imu frame : WBToolboxLibrary/wholeBodyModel/Kinematics/Forward Kinematics  frameName=FRAMES.imu  robotName=WBT_robotName  localName=WBT_modelName  wbiFile=WBT_wbiFilename  wbiList=WBT_wbiList
  link fixed with the seesaw : WBToolboxLibrary/wholeBodyModel/Kinematics/Forward Kinematics  frameName=FRAMES.fixedLink  robotName=WBT_robotName  localName=WBT_modelName  wbiFile=WBT_wbiFilename  wbiList=WBT_wbiList
  w_R_s : Outport
  s_omega : Outport  Port=2
  orientFromIMURobot : Outport  Port=3
  wires:
  Constant5/1 -> imu frame/1
  Inv\*/1 -> fromImuToHomogeousTransformFCN/1(imu_H_fixedLink), holder 1/1  "imu_H_fixedLink"
  imu frame/1 -> Inv\*/1
  Constant6/1 -> link fixed with the seesaw/1
  link fixed with the seesaw/1 -> Inv\*/2
  qj/1 -> link fixed with the seesaw/2, imu frame/2
  holder 1/1 -> fromImuToHomogeousTransformFCN/2(imu_H_fixedLink_0)
  holder 2/1 -> fromImuToHomogeousTransformFCN/3(imuRotation_0)
  neck position/1 -> Gain/1
  Selector1/1 -> Switch/1
  USE_IMU4EST_BASE1/1 -> Switch/2
  Switch/1 -> fromImuToHomogeousTransformFCN/6(neckPosition)
  Gain/1 -> Selector1/1
  Constant/1 -> Switch/3
  Select_rotation/1 -> fromImuToHomogeousTransformFCN/4(imuRotation), holder 2/1
  IMU_robot/1 -> Select_rotation/1, Select_velocity/1
  Gain1/1 -> s_omega/1
  fromImuToHomogeousTransformFCN/1(w_R_s) -> w_R_s/1
  Select_velocity/1 -> fromImuToHomogeousTransformFCN/5(wImu_omega)
  fromImuToHomogeousTransformFCN/3(orientFromIMURobot) -> orientFromIMURobot/1
  fromImuToHomogeousTransformFCN/2(s_omega) -> Gain1/1

== system controller/Robot and seesaw state/Seesaw orientation and angVelocity/Seesaw orientation and ang velocity from IMU seesaw ==
  IMU_seesaw : Inport
  Gain1 : Gain  Gain=pi/180
  Seesaw angular velocity with IMU seesaw : Subsystem
  Seesaw rotation with IMU_seesaw : Subsystem
  w_R_s : Outport
  s_omega : Outport  Port=2
  orientFromIMUSeesaw : Outport  Port=3
  wires:
  IMU_seesaw/1 -> Seesaw angular velocity with IMU seesaw/1(IMU_seesaw), Seesaw rotation with IMU_seesaw/1(IMU_seesaw)
  Seesaw angular velocity with IMU seesaw/1(s_omega) -> Gain1/1
  Seesaw rotation with IMU_seesaw/1(w_R_s) -> w_R_s/1
  Gain1/1 -> s_omega/1
  Seesaw rotation with IMU_seesaw/2(orientFromIMUSeesaw) -> orientFromIMUSeesaw/1

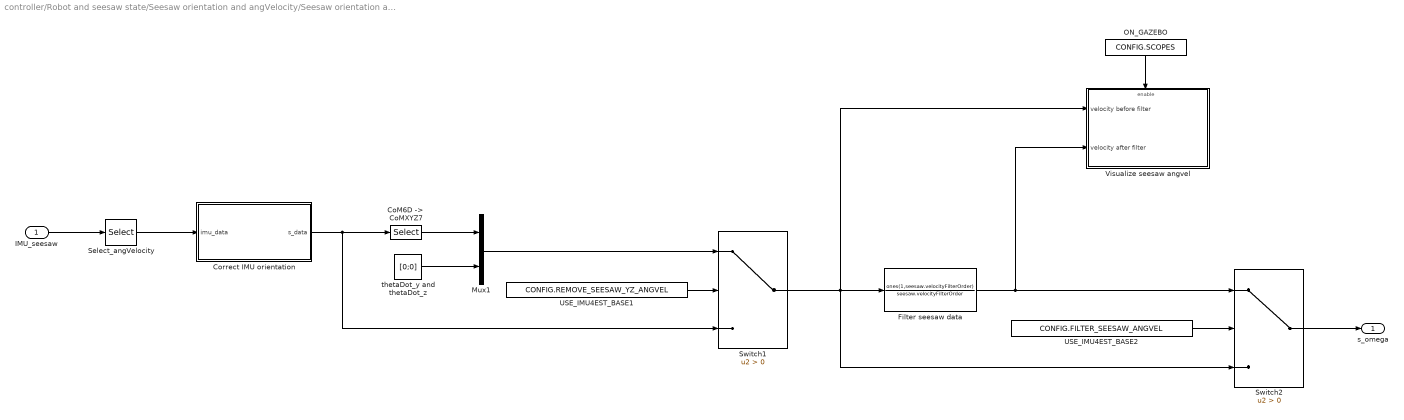
== system controller/Robot and seesaw state/Seesaw orientation and angVelocity/Seesaw orientation and ang velocity from IMU seesaw/Seesaw angular velocity with IMU seesaw ==
  IMU_seesaw : Inport
  "CoM6D ->  CoMXYZ7" : Selector  InputPortWidth=3  Indices=[1]
  Correct IMU orientation : MATLAB Function  TreatAsAtomicUnit=on
  Filter seesaw data : DiscreteFilter  Numerator=ones(1,seesaw.velocityFilterOrder)  Denominator=seesaw.velocityFilterOrder  SampleTime=CONFIG.TS
  Mux1 : Mux  Inputs=2
  "ON_GAZEBO " : Constant  Value=CONFIG.SCOPES
  Select_angVelocity : Selector  InputPortWidth=12  Indices=[7 8 9]
  Switch1 : Switch  Criteria=u2 > Threshold
  Switch2 : Switch  Criteria=u2 > Threshold
  USE_IMU4EST_BASE1 : Constant  Value=CONFIG.REMOVE_SEESAW_YZ_ANGVEL
  USE_IMU4EST_BASE2 : Constant  Value=CONFIG.FILTER_SEESAW_ANGVEL
  Visualize seesaw angvel : Subsystem
  thetaDot_y and thetaDot_z : Constant  Value=[0;0]
  s_omega : Outport
  wires:
  IMU_seesaw/1 -> Select_angVelocity/1
  USE_IMU4EST_BASE1/1 -> Switch1/2
  "CoM6D ->  CoMXYZ7"/1 -> Mux1/1
  thetaDot_y and thetaDot_z/1 -> Mux1/2
  Select_angVelocity/1 -> Correct IMU orientation/1(imu_data)
  Correct IMU orientation/1(s_data) -> "CoM6D ->  CoMXYZ7"/1, Switch1/3
  Mux1/1 -> Switch1/1
  USE_IMU4EST_BASE2/1 -> Switch2/2
  Switch2/1 -> s_omega/1
  Switch1/1 -> Visualize seesaw angvel/1(velocity before filter), Switch2/3, Filter seesaw data/1
  Filter seesaw data/1 -> Switch2/1, Visualize seesaw angvel/2(velocity after filter)
  "ON_GAZEBO "/1 -> Visualize seesaw angvel/Enable

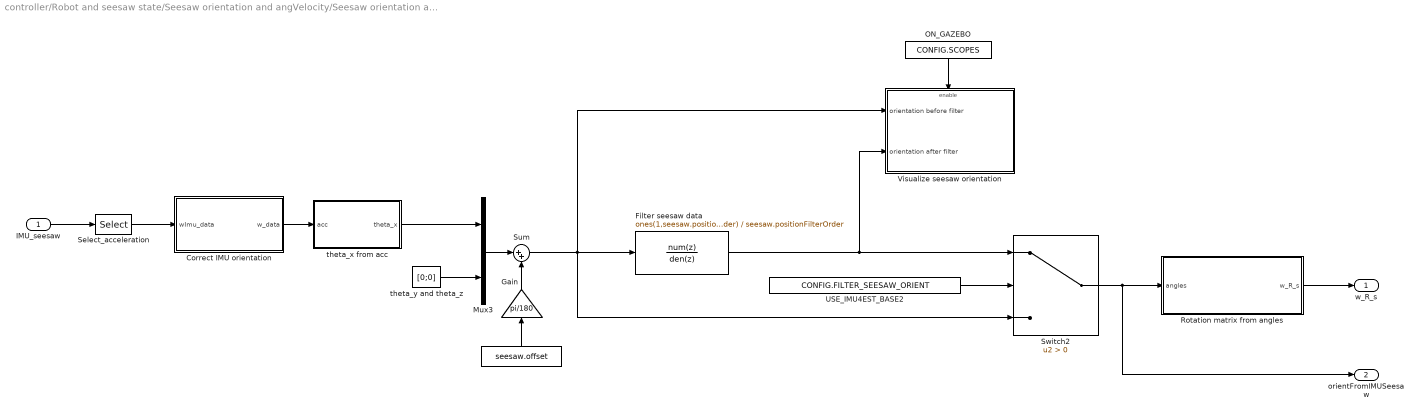
== system controller/Robot and seesaw state/Seesaw orientation and angVelocity/Seesaw orientation and ang velocity from IMU seesaw/Seesaw rotation with IMU_seesaw ==
  IMU_seesaw : Inport
  " " : Constant  Value=seesaw.offset
  Correct IMU orientation : MATLAB Function  TreatAsAtomicUnit=on
  Filter seesaw data : DiscreteFilter  Numerator=ones(1,seesaw.positionFilterOrder)  Denominator=seesaw.positionFilterOrder  SampleTime=CONFIG.TS
  Gain : Gain  Gain=pi/180
  Mux3 : Mux  Inputs=2
  "ON_GAZEBO " : Constant  Value=CONFIG.SCOPES
  Rotation matrix from angles : MATLAB Function  TreatAsAtomicUnit=on
  Select_acceleration : Selector  InputPortWidth=12  Indices=[4 5 6]
  Sum : Sum  Inputs=|++
  Switch2 : Switch  Criteria=u2 > Threshold
  USE_IMU4EST_BASE2 : Constant  Value=CONFIG.FILTER_SEESAW_ORIENT
  Visualize seesaw orientation : Subsystem
  theta_x from acc : MATLAB Function  TreatAsAtomicUnit=on
  theta_y and theta_z : Constant  Value=[0;0]
  w_R_s : Outport
  orientFromIMUSeesaw : Outport  Port=2
  wires:
  theta_x from acc/1(theta_x) -> Mux3/1
  theta_y and theta_z/1 -> Mux3/2
  Correct IMU orientation/1(w_data) -> theta_x from acc/1(acc)
  IMU_seesaw/1 -> Select_acceleration/1
  Select_acceleration/1 -> Correct IMU orientation/1(wImu_data)
  Rotation matrix from angles/1(w_R_s) -> w_R_s/1
  Mux3/1 -> Sum/1
  " "/1 -> Gain/1
  "ON_GAZEBO "/1 -> Visualize seesaw orientation/Enable
  USE_IMU4EST_BASE2/1 -> Switch2/2
  Switch2/1 -> Rotation matrix from angles/1(angles), orientFromIMUSeesaw/1
  Sum/1 -> Switch2/3, Visualize seesaw orientation/1(orientation before filter), Filter seesaw data/1
  Filter seesaw data/1 -> Visualize seesaw orientation/2(orientation after filter), Switch2/1
  Gain/1 -> Sum/2

== system controller/Robot and seesaw state/Seesaw orientation and angVelocity/Seesaw orientation and ang velocity from IMU seesaw/Seesaw angular velocity with IMU seesaw/Visualize seesaw angvel ==
  velocity before filter : Inport
  velocity after filter : Inport  Port=2
  Enable : EnablePort
  Mux : Mux  Inputs=2
  after filter : Scope
  before filter : Scope
  visualize delay : Scope
  wires:
  velocity before filter/1 -> Mux/1, before filter/1
  velocity after filter/1 -> Mux/2, after filter/1
  Mux/1 -> visualize delay/1

== system controller/Robot and seesaw state/Seesaw orientation and angVelocity/Seesaw orientation and ang velocity from IMU seesaw/Seesaw rotation with IMU_seesaw/Visualize seesaw orientation ==
  orientation before filter : Inport
  orientation after filter : Inport  Port=2
  Enable : EnablePort
  Mux : Mux  Inputs=2
  after filter : Scope
  before filter : Scope
  visualize delay : Scope
  wires:
  orientation before filter/1 -> Mux/1, before filter/1
  orientation after filter/1 -> Mux/2, after filter/1
  Mux/1 -> visualize delay/1

== matlab function Balancing controller and QP solver/balancingControlSeeSawFCN ==
  data: fNoQp output double; f_HDot output double; NA output double; t input double; state_0 input double; state input double; ConstraintsMatrix input double; bVectorConstraints input double; gain parameter double; reg parameter double; desired_x_dx_ddx_CoM input double; qjDes input double; seesaw parameter double; ROBOT_DOF input double; J input double; JCoM input double; JDot_nu input double; M input double; h input double; w_p_CoM input double; w_H_lSole input double; w_H_rSole input double; H input double; intHw input double; CONFIG parameter double; tauModel output double; Sigmaf_HDot output double; SigmaNA output double; HessianMatrixQP2Feet output double; gradientQP2Feet output double; ConstraintsMatrixQP2Feet output double; bVectorConstraintsQp2Feet output double; xCoM_seesaw input double; ddxCoM_seesaw output double; dxCoM_seesaw input double
function [fNoQp,f_HDot,NA,tauModel,Sigmaf_HDot,SigmaNA,...
          HessianMatrixQP2Feet,gradientQP2Feet,ConstraintsMatrixQP2Feet,bVectorConstraintsQp2Feet,ddxCoM_seesaw] = ...
          balancingControlSeesawFCN(t,state_0,state,ConstraintsMatrix,bVectorConstraints,gain,reg, ...
                                    desired_x_dx_ddx_CoM,qjDes,seesaw,ROBOT_DOF,...
                                    J,JCoM,JDot_nu,M,h,w_p_CoM,w_H_lSole,w_H_rSole,H,intHw,CONFIG,xCoM_seesaw,dxCoM_seesaw)

    % Organize the data in a structure to be compatible with the format of
    % the balancing controller
    
    % Robot data
    robot                              = struct;
    robot.M                            = M;
    robot.J                            = J;
    robot.JDot_nu                      = JDot_nu;  
    robot.h                            = h;
    robot.H                            = H;
    robot.intHw                        = intHw;
    robot.JCoM                         = JCoM;
    
    % Desired trajectory
    trajectory.qjDes                   = qjDes;
    trajectory.desired_x_dx_ddx_CoM    = desired_x_dx_ddx_CoM;
    
    % Robot and seesaw position and velocity
    [seesaw_pose, s_omega, q, nu]      = state_partitioning(state, length(ROBOT_DOF));
    w_R_s                              = rotationFromQuaternion(seesaw_pose(1:4));
    qj                                 = q(8:end);
    
    %% Balancing controller FCN
    [tauModel,Sigmaf_HDot,SigmaNA,ConstraintsMatrixQP2Feet,bVectorConstraintsQp2Feet,HessianMatrixQP2Feet,gradientQP2Feet,f_HDot,NA,ddxCoM_seesaw] = ...
        balancingController(w_R_s,s_omega,seesaw,robot,trajectory,gain,qj,nu,ConstraintsMatrix,bVectorConstraints, ...
                            w_H_lSole,w_H_rSole,w_p_CoM,reg,CONFIG,ROBOT_DOF,xCoM_seesaw,dxCoM_seesaw);

     % For visualization: retrieve the null space of contact forces (no QP)
     f0                = -pinvDamped(SigmaNA,reg.pinvTol)*(tauModel+Sigmaf_HDot);
     fNoQp             = f_HDot  + NA*f0;

end

== matlab function Robot CoM and joints references/trajectoryGeneratorCoM ==
  data: desired_x_dx_ddx_CoM output double; xCoM_0 input double; t input double; referenceParams input double; directionOfOscillation input double; noOscillationTime input double
function desired_x_dx_ddx_CoM = trajectoryGeneratorFCN(xCoM_0, t, referenceParams, directionOfOscillation, noOscillationTime)

desired_x_dx_ddx_CoM = trajectoryGenerator(xCoM_0, t, referenceParams, directionOfOscillation, noOscillationTime);

end

== matlab function Robot and seesaw state/Seesaw orientation and angVelocity/Seesaw orientation and ang velocity from IMU robot/fromImuToHomogeousTransformFCN ==
  data: imu_H_fixedLink input double; imu_H_fixedLink_0 input double; imuRotation_0 input double; imuRotation input double; wImu_omega input double; neckPosition input double; w_R_s output double; CONFIG parameter double; s_omega output double; orientFromIMURobot output double; seesaw parameter double
function [w_R_s,s_omega,orientFromIMURobot] = fromIMUtoWorldFrameFCN ...
                                              (imu_H_fixedLink,imu_H_fixedLink_0,imuRotation_0,imuRotation,wImu_omega,neckPosition,CONFIG,seesaw)

[w_R_s,s_omega,orientFromIMURobot] = fromIMUtoWorldFrame ...
                                     (imu_H_fixedLink,imu_H_fixedLink_0,imuRotation_0,imuRotation,wImu_omega,neckPosition,CONFIG,seesaw);
 
end

== matlab function Robot and seesaw state/Seesaw orientation and angVelocity/Seesaw orientation and ang velocity from IMU seesaw/Seesaw angular velocity with IMU seesaw/Correct IMU orientation ==
  data: imu_data input double; s_data output double; seesaw parameter double
function s_data = rotateImuWorldFrameFCN(imu_data,seesaw)

% The angular velocity is expressed in a frame attached to the IMU (imu frame), not 
% in wImu frame. Then, this trasformation is giving the angular velocity expressed 
% in the seesaw frame, not in world frame.
s_data = rotateImuWorldFrame(imu_data,seesaw);

end

== matlab function Robot and seesaw state/Seesaw orientation and angVelocity/Seesaw orientation and ang velocity from IMU seesaw/Seesaw rotation with IMU_seesaw/Correct IMU orientation ==
  data: wImu_data input double; w_data output double; seesaw parameter double
function w_data = rotateImuWorldFrameFCN(wImu_data,seesaw)

w_data = rotateImuWorldFrame(wImu_data,seesaw);

end

== matlab function Robot and seesaw state/Seesaw orientation and angVelocity/Seesaw orientation and ang velocity from IMU seesaw/Seesaw rotation with IMU_seesaw/theta_x from acc ==
  data: acc input double; theta_x output double
function theta_x = arctangent(acc)

% theta_x (seesaw roll) in radians
theta_x = atan2(acc(2),acc(3));

end

== matlab function Robot and seesaw state/Seesaw orientation and angVelocity/Seesaw orientation and ang velocity from IMU seesaw/Seesaw rotation with IMU_seesaw/Rotation matrix from angles ==
  data: angles input double; w_R_s output double
function w_R_s = rotationMatrixFromAngles(angles)

% See http://wiki.icub.org/images/8/82/XsensMtx.pdf page 12
w_R_s = rotz(angles(3))*roty(angles(2))*rotx(angles(1));

end

== matlab function Robot and seesaw state/Compute w_H_b and Qs /MATLAB Function ==
  data: Qs output double; w_R_s input double
function Qs = quaternionFromRotationMatrixFCN(w_R_s)

Qs = quaternionFromRotationMatrix(w_R_s);

end

== matlab function Robot and seesaw state/Compute base velocity/evaluateBaseVelocity ==
  data: v_base output double; J_fixedLink input double; w_R_s input double; dqj input double; s_omega input double; seesaw parameter double; reg parameter double
function v_base  = computeBaseVelocityFCN(J_fixedLink,w_R_s,dqj,s_omega,seesaw,reg)

    v_base = computeBaseVelocity(J_fixedLink,w_R_s,dqj,s_omega,seesaw,reg);

end

== matlab function Robot and seesaw state/Compute w_H_b and Qs /Compute w_H_fixedLink/fixedLink w.r.t the world frame ==
  data: w_R_s input double; w_H_fixedLink output double; seesaw parameter double
function w_H_fixedLink = computeTransFromFixedLinkToWorldFCN(w_R_s,seesaw)

w_H_fixedLink = computeTransFromFixedLinkToWorld(w_R_s,seesaw);

end

== matlab function Balancing controller and QP solver/integral of Hw /MATLAB Function ==
  data: qjErr input double; JL input double; JR input double; vbEquivalent output double; reg parameter double; activeFeetConstraints input double
function vbEquivalent = generateReferencesForH(qjErr,JL,JR,reg,activeFeetConstraints)

% The approximation of integral of angular momentum is given by:
%
%    H_approx = JG(qRef)*(qj-qjDes)
%
% It is assumed here that one of the feet is always on ground at time t=0
% 
if activeFeetConstraints(1) == 1
    
    pinvJb             = (transpose(JL(:,1:6))*JL(:,1:6) + reg.pinvTolVb*eye(6))\transpose(JL(:,1:6));
    vbEquivalent       = -pinvJb*JL(:,7:end)*qjErr;
else
    
    pinvJb             = (transpose(JR(:,1:6))*JR(:,1:6) + reg.pinvTolVb*eye(6))\transpose(JR(:,1:6));
    vbEquivalent       = -pinvJb*JR(:,7:end)*qjErr;
end
end
